simulink model "FOCModel"  (R2025b)
settings: Solver=VariableStepAuto  StartTime=0.0  StopTime=10.0  RelTol=1e-3
libraries: autolibim x2, eeAsmDtcSvm x1, eeAsmFieldOrientedControl x1

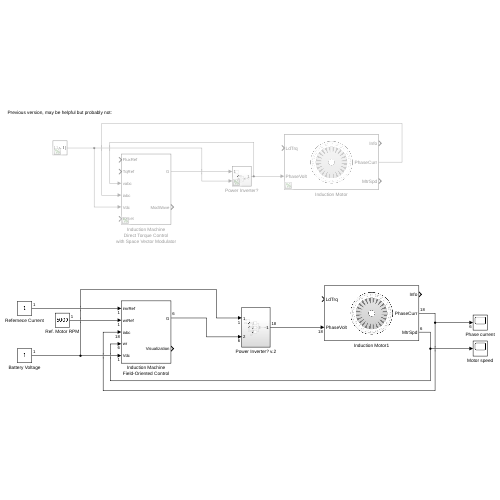
[thumbnail: Simulink's stored preview of the top-level diagram]
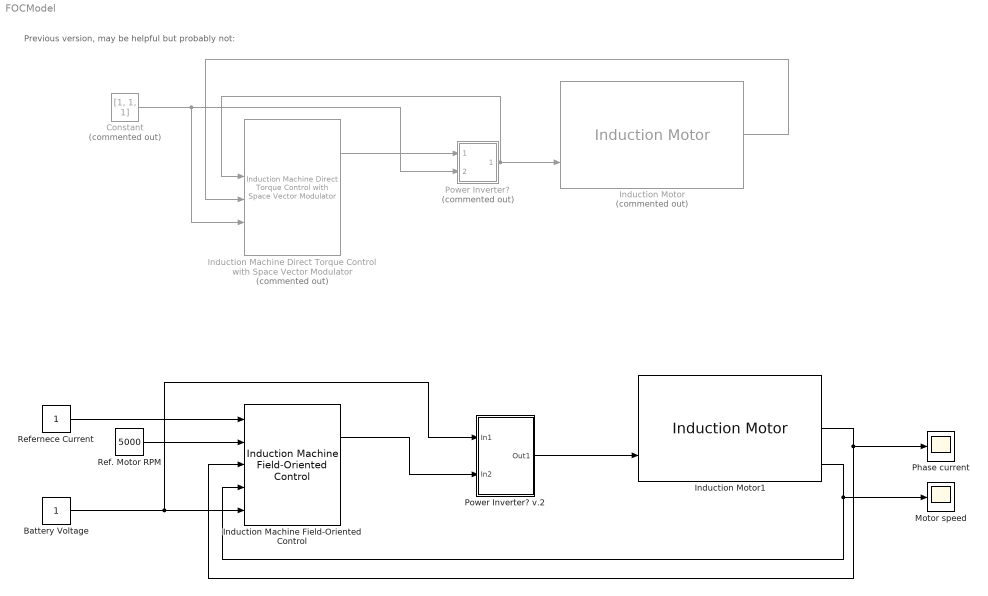
== system FOCModel ==
  note: Previous version, may be helpful but probably not:
  Battery Voltage : Constant
  Constant : Constant  Commented=on  Value=[1, 1, 1]
  Induction Machine Direct Torque Control with Space Vector Modulator : eeAsmDtcSvm/Induction Machine Direct Torque Control with Space Vector Modulator  Commented=on  Rs=0.25  p=1  Vdc_on=300  Ts=5e-6  Tsc=5e-5  fsw=1000  Kp_flux=150  Ki_flux=3000  Kaw_flux=1  Kp_tq=1  Ki_tq=50  Kaw_tq=1  AxisPrio=Q-axis
      settings: LibrarySourceBlock=|
      | ee_sl_lib/Induction Machine
      | Control/Induction Machine
      | Direct Torque Control
      | with Space Vector Modulator
  Induction Machine Field-Oriented Control : eeAsmFieldOrientedControl/Induction Machine Field-Oriented Control  Vn=550  fn=60  Rr=0.01  Llr=0.06  Lm=2.7  Tc=1e-4  Vdc_on=500  Ts=5e-6  Tsc=5e-5  Kp_imr=10  Ki_imr=1000  Kaw_imr=1000  Kp_wr=10  Ki_wr=1000  Kaw_wr=1000  id_max=2  iq_max=2  AxisAlignment=Q-axis  Kp_id=1  Ki_id=100  Kaw_id=1  Kp_iq=1  Ki_iq=100  Kaw_iq=1  AxisPrio=Q-axis  CPWMMode=SPWM: sinusoidal PWM  fsw=1000
      settings: SamplingMode=Natural
      settings: LibrarySourceBlock=|
      | ee_sl_lib/Induction Machine
      | Control/Induction Machine
      | Field-Oriented Control
  Induction Motor : autolibim/Induction Motor  Commented=on  sim_type=Continuous  Ts=0.001  port_config=Torque  P=2  Zs=[1.77 0.0139]  Zr="[1.34  0.0121]"  Lm=0.3687  mechanical=[0.001 0 0]  theta_init=0  omega_init=0  RefBlkName='autolibim/Induction Motor'  aMode=1
      settings: LibrarySourceBlock=autolibemachines/Induction Motor
  Induction Motor1 : autolibim/Induction Motor  sim_type=Continuous  Ts=0.001  port_config=Torque  P=11  Zs=[1.77 0.0139]  Zr="[1.34  0.0121]"  Lm=0.3687  mechanical=[0.001 0 0]  theta_init=0  omega_init=0  RefBlkName='autolibim/Induction Motor'  aMode=1
      settings: LibrarySourceBlock=autolibemachines/Induction Motor
  Motor speed : Scope
  Phase current : Scope
  Power Inverter? : Subsystem  Commented=on
  Power Inverter? v.2 : Subsystem
  Ref. Motor RPM : Constant  Value=5000
  Refernece Current : Constant
  wires:
  Induction Machine Direct Torque Control with Space Vector Modulator/1 -> Power Inverter?/1(In1)
  Power Inverter?/1(Out1) -> Induction Machine Direct Torque Control with Space Vector Modulator/3, Induction Motor/2
  Induction Motor/2 -> Induction Machine Direct Torque Control with Space Vector Modulator/4
  Constant/1 -> Induction Machine Direct Torque Control with Space Vector Modulator/5, Power Inverter?/2(In2)
  Battery Voltage/1 -> Induction Machine Field-Oriented Control/5, Power Inverter? v.2/1(In1)
  Induction Machine Field-Oriented Control/1 -> Power Inverter? v.2/2(In2)
  Power Inverter? v.2/1(Out1) -> Induction Motor1/2
  Induction Motor1/2 -> Phase current/1, Induction Machine Field-Oriented Control/3
  Refernece Current/1 -> Induction Machine Field-Oriented Control/1
  Induction Motor1/3 -> Motor speed/1, Induction Machine Field-Oriented Control/4
  Ref. Motor RPM/1 -> Induction Machine Field-Oriented Control/2

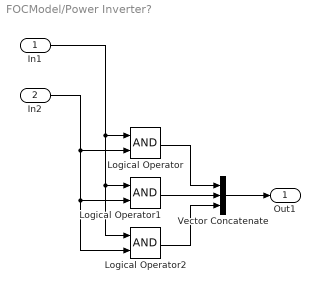
== system FOCModel/Power Inverter? ==
  In1 : Inport
  In2 : Inport  Port=2
  Logical Operator : Logic  AllPortsSameDT=off  OutDataTypeStr=boolean
  Logical Operator1 : Logic  AllPortsSameDT=off  OutDataTypeStr=boolean
  Logical Operator2 : Logic  AllPortsSameDT=off  OutDataTypeStr=boolean
  Vector Concatenate : Concatenate  NumInputs=3
  Out1 : Outport
  wires:
  Vector Concatenate/1 -> Out1/1
  Logical Operator1/1 -> Vector Concatenate/2
  Logical Operator/1 -> Vector Concatenate/1
  In1/1 -> Logical Operator/1, Logical Operator1/1, Logical Operator2/1
  In2/1 -> Logical Operator1/2, Logical Operator2/2, Logical Operator/2
  Logical Operator2/1 -> Vector Concatenate/3

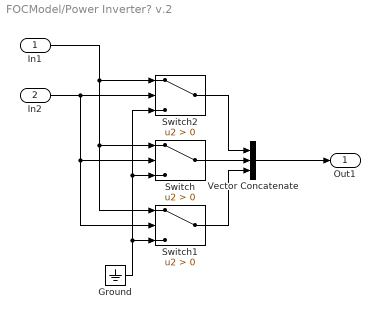
== system FOCModel/Power Inverter? v.2 ==
  In1 : Inport
  In2 : Inport  Port=2
  Ground : Ground
  Switch : Switch  Criteria=u2 > Threshold  SaturateOnIntegerOverflow=off  InputSameDT=off
  Switch1 : Switch  Criteria=u2 > Threshold  SaturateOnIntegerOverflow=off  InputSameDT=off
  Switch2 : Switch  Criteria=u2 > Threshold  SaturateOnIntegerOverflow=off  InputSameDT=off
  Vector Concatenate : Concatenate  NumInputs=3
  Out1 : Outport
  wires:
  In1/1 -> Switch1/1, Switch/1, Switch2/1
  Ground/1 -> Switch2/3, Switch/3, Switch1/3
  In2/1 -> Switch1/2, Switch/2, Switch2/2
  Switch1/1 -> Vector Concatenate/3
  Switch/1 -> Vector Concatenate/2
  Switch2/1 -> Vector Concatenate/1
  Vector Concatenate/1 -> Out1/1
